simulink model "Clutch_LockUp"  (R2020b)
settings: Solver=VariableStepAuto  StartTime=0.0  StopTime=10.0  RelTol=1e-3
values from neighbouring files (symbols this model uses):
  be = 2.0    [Clutch_Data_Dict.sldd]
  bv = 1.0    [Clutch_Data_Dict.sldd]
  Fn = 0.0 1.0 2.0 3.0 4.0 5.0 6.0 7.0 8.0 9.0 10.0 0.0 0.8 1.6 1.6 1.6 1.6 0.8 0.0 0.0 0.0 0.0    [Clutch_Data_Dict.sldd]
  Ie = 1.0    [Clutch_Data_Dict.sldd]
  Iv = 5.0    [Clutch_Data_Dict.sldd]
  muk = 1.0    [Clutch_Data_Dict.sldd]
  mus = 1.5    [Clutch_Data_Dict.sldd]
  R = 1.0    [Clutch_Data_Dict.sldd]
settings Model: DataDictionary=Clutch_Data_Dict.sldd  Creator=vijay jagtap  LastModifiedBy=vijay jagtap
settings SolverCC: ZeroCrossAlgorithm=Adaptive
settings DebuggingCC: IgnoredZcDiagnostic=none

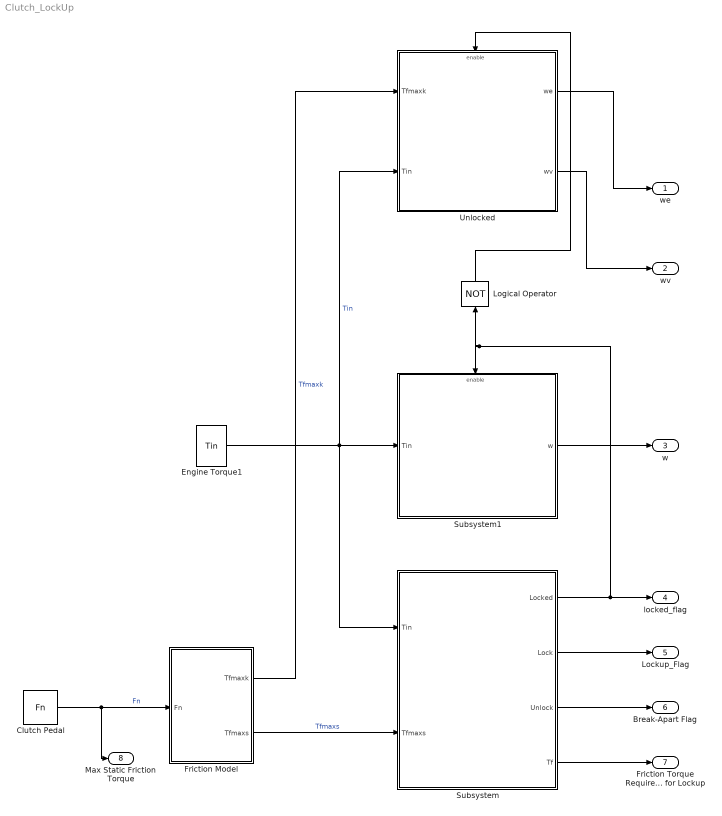
== system Clutch_LockUp ==
  Clutch Pedal : Constant  Value=Fn
  Engine Torque1 : FromWorkspace  VariableName=Tin  ZeroCross=off
  Friction Model : Subsystem
  Logical Operator : Logic  Operator=NOT  AllPortsSameDT=off  OutDataTypeStr=boolean
  Subsystem : Subsystem
  Subsystem1 : Subsystem
  Unlocked : Subsystem
  we : Outport
  wv : Outport  Port=2
  w : Outport  Port=3
  locked_flag : Outport  Port=4
  Lockup_Flag : Outport  Port=5
  Break-Apart Flag : Outport  Port=6
  Friction Torque Required for Lockup : Outport  Port=7
  Max Static Friction Torque : Outport  Port=8
  wires:
  Clutch Pedal/1 -> Max Static Friction Torque/1, Friction Model/1(Fn)  "Fn"
  Friction Model/2(Tfmaxs) -> Subsystem/2(Tfmaxs)  "Tfmaxs"
  Engine Torque1/1 -> Unlocked/2(Tin), Subsystem1/1(Tin), Subsystem/1(Tin)  "Tin"
  Friction Model/1(Tfmaxk) -> Unlocked/1(Tfmaxk)  "Tfmaxk"
  Subsystem/1(Locked) -> Subsystem1/Enable, Logical Operator/1, locked_flag/1
  Subsystem/2(Lock) -> Lockup_Flag/1
  Subsystem/3(Unlock) -> Break-Apart Flag/1
  Subsystem/4(Tf) -> Friction Torque Required for Lockup/1
  Subsystem1/1(w) -> w/1
  Unlocked/2(wv) -> wv/1
  Unlocked/1(we) -> we/1
  Logical Operator/1 -> Unlocked/Enable

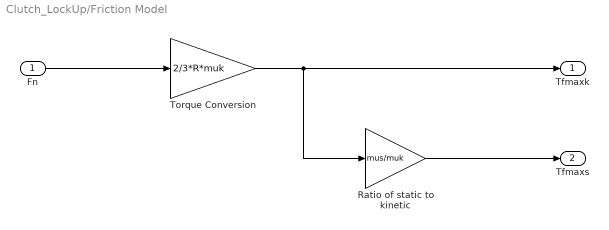
== system Clutch_LockUp/Friction Model ==
  Fn : Inport
  Ratio of static to kinetic : Gain  Gain=mus/muk  SaturateOnIntegerOverflow=on  OutDataTypeStr=Inherit: Same as input  ParamDataTypeStr=Inherit: Same as input
  Torque Conversion : Gain  Gain=2/3*R*muk  SaturateOnIntegerOverflow=on  OutDataTypeStr=Inherit: Same as input  ParamDataTypeStr=Inherit: Same as input
  Tfmaxk : Outport  InitialOutput=0  VectorParamsAs1DForOutWhenUnconnected=off
  Tfmaxs : Outport  Port=2  InitialOutput=0  VectorParamsAs1DForOutWhenUnconnected=off
  wires:
  Torque Conversion/1 -> Tfmaxk/1, Ratio of static to kinetic/1
  Fn/1 -> Torque Conversion/1
  Ratio of static to kinetic/1 -> Tfmaxs/1

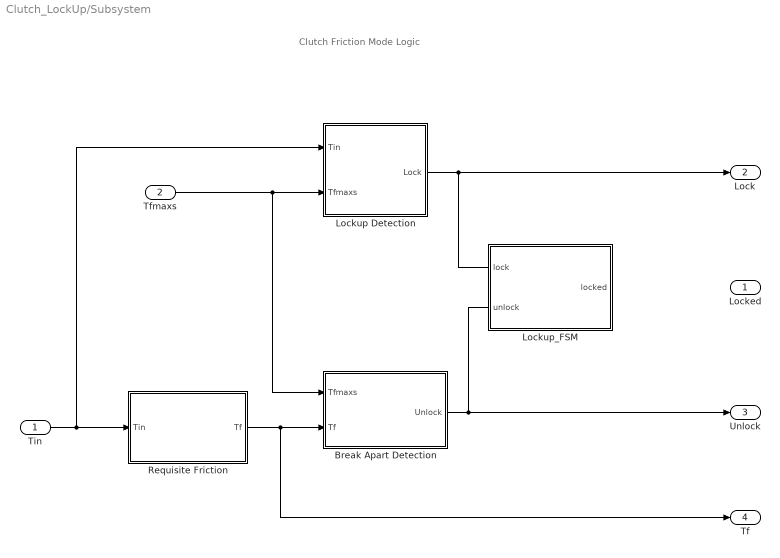
== system Clutch_LockUp/Subsystem ==
  note: Clutch Friction Mode Logic
  Tin : Inport
  Tfmaxs : Inport  Port=2
  Break Apart Detection : Subsystem
  Lockup Detection : Subsystem
  Lockup_FSM : Subsystem
  Requisite Friction : Subsystem
  Locked : Outport
  Lock : Outport  Port=2
  Unlock : Outport  Port=3
  Tf : Outport  Port=4
  wires:
  Requisite Friction/1(Tf) -> Tf/1, Break Apart Detection/2(Tf)
  Break Apart Detection/1(Unlock) -> Unlock/1
  Lockup Detection/1(Lock) -> Lock/1
  Tin/1 -> Lockup Detection/1(Tin), Requisite Friction/1(Tin)
  Tfmaxs/1 -> Break Apart Detection/1(Tfmaxs), Lockup Detection/2(Tfmaxs)
  ? -> Locked/1

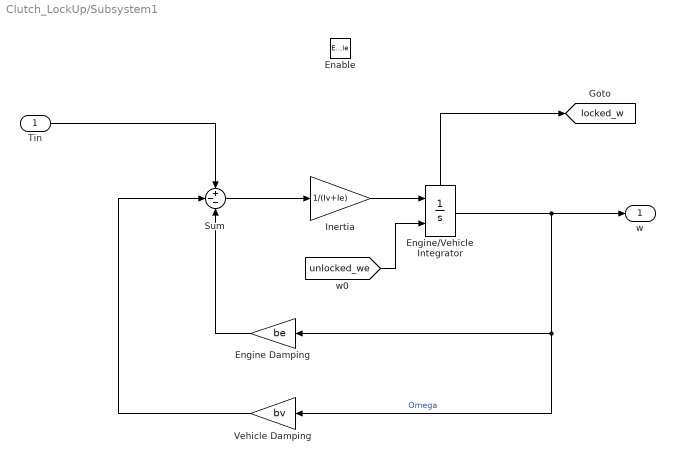
== system Clutch_LockUp/Subsystem1 ==
  Tin : Inport
  Enable : EnablePort  StatesWhenEnabling=reset
  Engine Damping : Gain  Gain=be  SaturateOnIntegerOverflow=on  OutDataTypeStr=Inherit: Same as input  ParamDataTypeStr=Inherit: Same as input
  Engine/Vehicle Integrator : Integrator  InitialConditionSource=external  ShowStatePort=on
  Inertia : Gain  Gain=1/(Iv+Ie)  SaturateOnIntegerOverflow=on  OutDataTypeStr=Inherit: Same as input  ParamDataTypeStr=Inherit: Same as input
  Sum : Sum  Inputs=+--  InputSameDT=on  SaturateOnIntegerOverflow=on  OutDataTypeStr=Inherit: Same as first input
  Vehicle Damping : Gain  Gain=bv  SaturateOnIntegerOverflow=on  OutDataTypeStr=Inherit: Same as input  ParamDataTypeStr=Inherit: Same as input
  w : Outport  InitialOutput=0  VectorParamsAs1DForOutWhenUnconnected=off
  tag scope: locked_w=global
  wires:
  [unlocked_we] -> Engine/Vehicle Integrator/2
  Engine/Vehicle Integrator/1 -> Engine Damping/1, Vehicle Damping/1, w/1  "Omega"
  Engine/Vehicle Integrator/State -> [locked_w]
  Vehicle Damping/1 -> Sum/2
  Sum/1 -> Inertia/1
  Tin/1 -> Sum/1
  Engine Damping/1 -> Sum/3
  Inertia/1 -> Engine/Vehicle Integrator/1

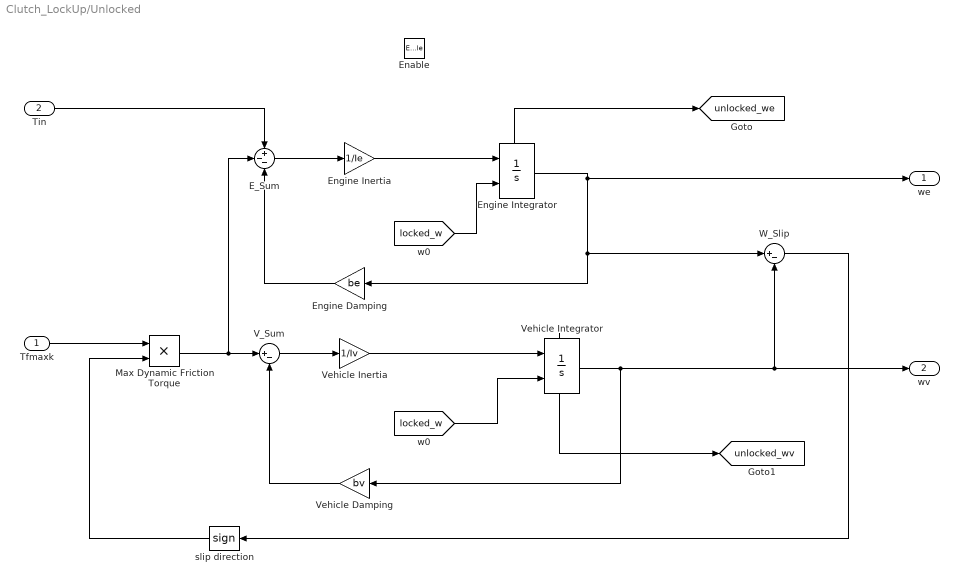
== system Clutch_LockUp/Unlocked ==
  Tfmaxk : Inport
  Tin : Inport  Port=2
  Enable : EnablePort  StatesWhenEnabling=reset
  E_Sum : Sum  Inputs=+--  InputSameDT=on  SaturateOnIntegerOverflow=on  OutDataTypeStr=Inherit: Same as first input
  Engine Damping : Gain  Gain=be  SaturateOnIntegerOverflow=on  OutDataTypeStr=Inherit: Same as input  ParamDataTypeStr=Inherit: Same as input
  Engine Inertia : Gain  Gain=1/Ie  SaturateOnIntegerOverflow=on  OutDataTypeStr=Inherit: Same as input  ParamDataTypeStr=Inherit: Same as input
  Engine Integrator : Integrator  InitialConditionSource=external  ShowStatePort=on
  Max Dynamic Friction Torque : Product  InputSameDT=on  RndMeth=Zero  SaturateOnIntegerOverflow=on  OutDataTypeStr=Inherit: Same as first input
  V_Sum : Sum  Inputs=|+-  InputSameDT=on  SaturateOnIntegerOverflow=on  OutDataTypeStr=Inherit: Same as first input
  Vehicle Damping : Gain  Gain=bv  SaturateOnIntegerOverflow=on  OutDataTypeStr=Inherit: Same as input  ParamDataTypeStr=Inherit: Same as input
  Vehicle Inertia : Gain  Gain=1/Iv  SaturateOnIntegerOverflow=on  OutDataTypeStr=Inherit: Same as input  ParamDataTypeStr=Inherit: Same as input
  Vehicle Integrator : Integrator  InitialConditionSource=external  ShowStatePort=on
  W_Slip : Sum  Inputs=|+-  InputSameDT=on  SaturateOnIntegerOverflow=on  OutDataTypeStr=Inherit: Same as first input
  slip direction : Signum
  we : Outport  InitialOutput=0  VectorParamsAs1DForOutWhenUnconnected=off
  wv : Outport  Port=2  InitialOutput=0  VectorParamsAs1DForOutWhenUnconnected=off
  tag scope: unlocked_we=global, unlocked_wv=global
  wires:
  E_Sum/1 -> Engine Inertia/1
  V_Sum/1 -> Vehicle Inertia/1
  [locked_w] -> Engine Integrator/2
  Max Dynamic Friction Torque/1 -> V_Sum/1, E_Sum/2
  Engine Integrator/State -> [unlocked_we]
  [locked_w] -> Vehicle Integrator/2
  Vehicle Integrator/State -> [unlocked_wv]
  slip direction/1 -> Max Dynamic Friction Torque/2
  Vehicle Integrator/1 -> wv/1, W_Slip/2, Vehicle Damping/1
  Vehicle Inertia/1 -> Vehicle Integrator/1
  Engine Integrator/1 -> we/1, Engine Damping/1, W_Slip/1
  Tfmaxk/1 -> Max Dynamic Friction Torque/1
  Engine Inertia/1 -> Engine Integrator/1
  W_Slip/1 -> slip direction/1
  Engine Damping/1 -> E_Sum/3
  Vehicle Damping/1 -> V_Sum/2
  Tin/1 -> E_Sum/1

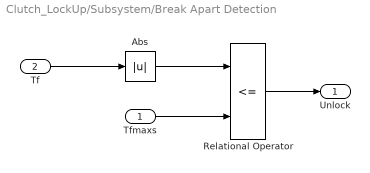
== system Clutch_LockUp/Subsystem/Break Apart Detection ==
  Tfmaxs : Inport
  Tf : Inport  Port=2
  Abs : Abs
  Relational Operator : RelationalOperator  Operator=<=  OutDataTypeStr=boolean  RndMeth=Simplest
  Unlock : Outport
  wires:
  Abs/1 -> Relational Operator/1
  Tfmaxs/1 -> Relational Operator/2
  Tf/1 -> Abs/1
  Relational Operator/1 -> Unlock/1

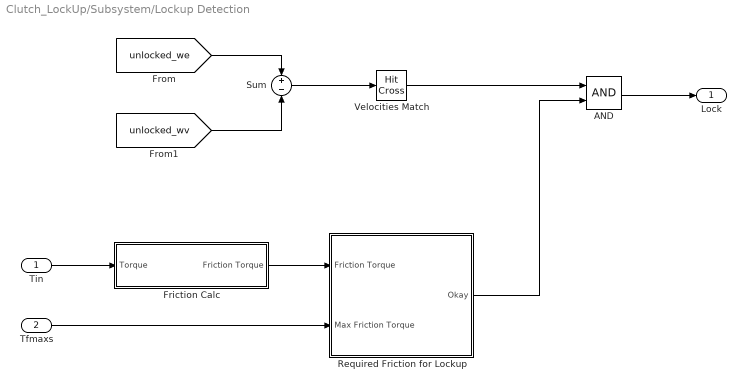
== system Clutch_LockUp/Subsystem/Lockup Detection ==
  Tin : Inport
  Tfmaxs : Inport  Port=2
  AND : Logic  AllPortsSameDT=off  OutDataTypeStr=boolean
  Friction Calc : Subsystem
  Required Friction for Lockup : Subsystem
  Sum : Sum  Inputs=+-
  Velocities Match : HitCross
  Lock : Outport
  wires:
  Friction Calc/1(Friction Torque) -> Required Friction for Lockup/1(Friction Torque)
  [unlocked_we] -> Sum/1
  [unlocked_wv] -> Sum/2
  Tin/1 -> Friction Calc/1(Torque)
  Tfmaxs/1 -> Required Friction for Lockup/2(Max Friction Torque)
  Sum/1 -> Velocities Match/1
  Velocities Match/1 -> AND/1
  Required Friction for Lockup/1(Okay) -> AND/2
  AND/1 -> Lock/1

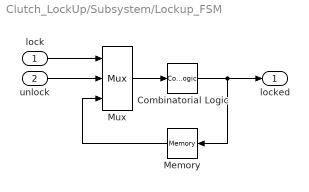
== system Clutch_LockUp/Subsystem/Lockup_FSM ==
  lock : Inport
  unlock : Inport  Port=2
  Combinatorial Logic : CombinatorialLogic  TruthTable=[0;1;0;0;1;1;1;0]
  Memory : Memory
  Mux : Mux  Inputs=3
  locked : Outport  InitialOutput=0  VectorParamsAs1DForOutWhenUnconnected=off
  wires:
  lock/1 -> Mux/1
  Mux/1 -> Combinatorial Logic/1
  Combinatorial Logic/1 -> locked/1, Memory/1
  Memory/1 -> Mux/3
  unlock/1 -> Mux/2

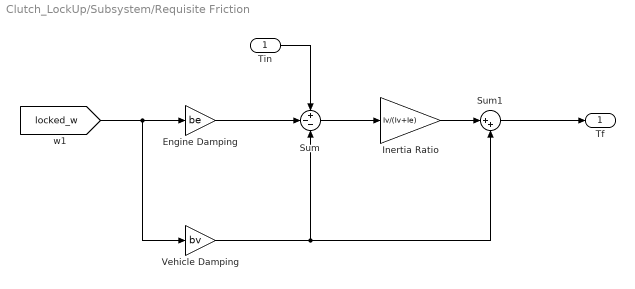
== system Clutch_LockUp/Subsystem/Requisite Friction ==
  Tin : Inport
  Engine Damping : Gain  Gain=be
  Inertia Ratio : Gain  Gain=Iv/(Iv+Ie)
  Sum : Sum  Inputs=+--
  Sum1 : Sum  Inputs=|++
  Vehicle Damping : Gain  Gain=bv
  Tf : Outport
  wires:
  Vehicle Damping/1 -> Sum1/2, Sum/3
  Engine Damping/1 -> Sum/2
  Tin/1 -> Sum/1
  [locked_w] -> Vehicle Damping/1, Engine Damping/1
  Sum1/1 -> Tf/1
  Inertia Ratio/1 -> Sum1/1
  Sum/1 -> Inertia Ratio/1

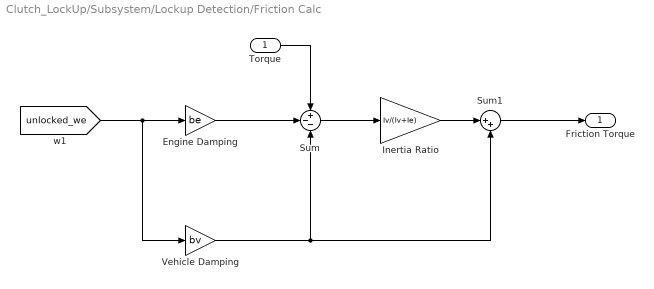
== system Clutch_LockUp/Subsystem/Lockup Detection/Friction Calc ==
  Torque : Inport
  Engine Damping : Gain  Gain=be
  Inertia Ratio : Gain  Gain=Iv/(Iv+Ie)
  Sum : Sum  Inputs=+--
  Sum1 : Sum  Inputs=|++
  Vehicle Damping : Gain  Gain=bv
  Friction Torque : Outport
  wires:
  Engine Damping/1 -> Sum/2
  Sum/1 -> Inertia Ratio/1
  [unlocked_we] -> Vehicle Damping/1, Engine Damping/1
  Vehicle Damping/1 -> Sum1/2, Sum/3
  Torque/1 -> Sum/1
  Inertia Ratio/1 -> Sum1/1
  Sum1/1 -> Friction Torque/1

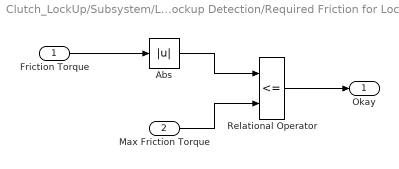
== system Clutch_LockUp/Subsystem/Lockup Detection/Required Friction for Lockup ==
  Friction Torque : Inport
  Max Friction Torque : Inport  Port=2
  Abs : Abs  SaturateOnIntegerOverflow=on
  Relational Operator : RelationalOperator  Operator=<=  OutDataTypeStr=boolean  RndMeth=Nearest
  Okay : Outport
  wires:
  Abs/1 -> Relational Operator/1
  Friction Torque/1 -> Abs/1
  Max Friction Torque/1 -> Relational Operator/2
  Relational Operator/1 -> Okay/1
